simulink model "s298637_sim"  (R2024a)
settings: Solver=VariableStepAuto  StartTime=0.0  StopTime=10.0  RelTol=1e-3
values from neighbouring files (symbols this model uses):
  dda = 0    [exsim.m]    (also in s298637.mat = 0.4)
  ddt = 1    [exsim.m]    (also in s298637.mat = 0)
  rho = 0    [exsim.m]    (also in s298637.mat)
  T_s = 0.015    [exsim.m]    (also in s298637.mat)
  wdt = 100    [exsim.m]    (also in s298637.mat)
libraries: cstblocks x2
settings Model: Creator=PC  LastModifiedBy=PC

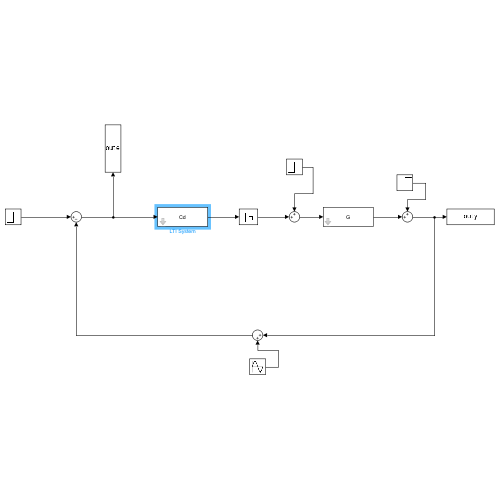
[thumbnail: Simulink's stored preview of the top-level diagram]
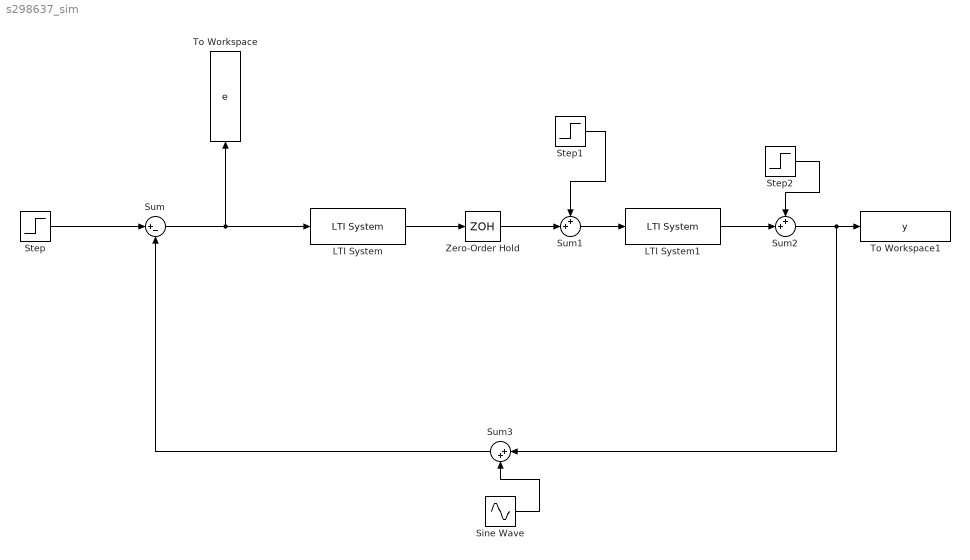
== system s298637_sim ==
  LTI System : cstblocks/LTI System  sys=Cd  IC=[]  PadeOrder=0
  LTI System1 : cstblocks/LTI System  sys=G  IC=[]  PadeOrder=0
  Sine Wave : Sin  Amplitude=ddt  Frequency=wdt  SampleTime=0
  Step : Step  Time=0  After=rho  SampleTime=0
  Step1 : Step  Time=0  After=dda  SampleTime=0
  Step2 : Step  Time=0  After=0  SampleTime=0
  Sum : Sum  Inputs=|+-
  Sum1 : Sum  Inputs=++|
  Sum2 : Sum  Inputs=++|
  Sum3 : Sum  Inputs=|++
  To Workspace : ToWorkspace  VariableName=e  SaveFormat=Timeseries  SampleTime=-1
  To Workspace1 : ToWorkspace  VariableName=y  SaveFormat=Timeseries  SampleTime=-1
  Zero-Order Hold : ZeroOrderHold  SampleTime=T_s
  wires:
  Step/1 -> Sum/1
  Sum/1 -> LTI System/1, To Workspace/1
  LTI System/1 -> Zero-Order Hold/1
  Zero-Order Hold/1 -> Sum1/2
  Sum1/1 -> LTI System1/1
  Sum2/1 -> Sum3/1, To Workspace1/1
  Sum3/1 -> Sum/2
  Step1/1 -> Sum1/1
  LTI System1/1 -> Sum2/2
  Step2/1 -> Sum2/1
  Sine Wave/1 -> Sum3/2
